simulink model "robot"  (R2024a)
settings: Solver=FixedStepDiscrete  StartTime=0.0  StopTime=inf  FixedStep=0.01  RelTol=1e-3
values from neighbouring files (symbols this model uses):
  markParams = struct()    [markParameters.m]
  mazeForSim = evalin('base',mapVar)    [mySetupRobotSim.m]
  robotParams = struct()    [robotParameters.m]
undefined symbols (not defined in the file or in its folder): D, DiscIntNeverNeededParam, InputPWM, Ts, uDelay, wheelMotorModel, WheelSpeed, xinit, yDelay
libraries: simulink x20, cstblocks x2, simulink_extras x1, mobileRoboticsTrainingLib x1
settings Model: Creator=ngcoya  LastModifiedBy=ngcoya
settings DataIOCC: ExternalInput=maze

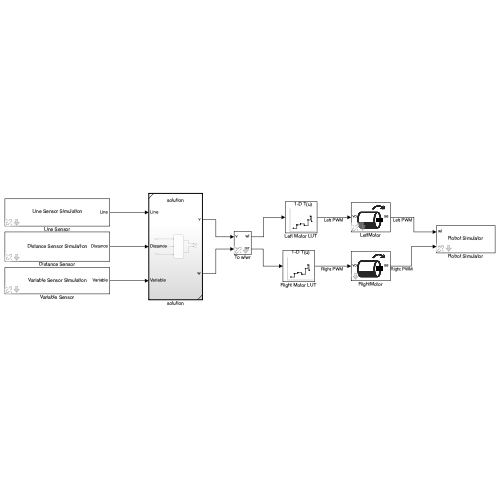
[thumbnail: Simulink's stored preview of the top-level diagram]
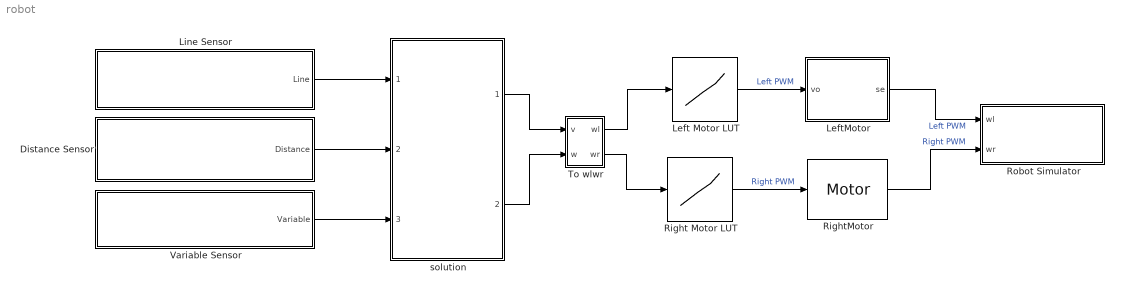
== system robot ==
  Distance Sensor : Subsystem  AncestorBlock=mobileRoboticsTrainingLib/Line Sensor  mask(Line Sensor Simulation){mapVariable=mazeForSim}
      mask prompts: mapVariable "Map Variable"
      mask help: Use a simulation map to compute line sensor values based on robot position and sensor offsets.
      mask Help: web('Line Sensor Simulation.htm')
      mask DialogControl DescTextVar Prompt: Use a simulation map to compute distance sensor values based on robot position and sensor parameters.
      mask DialogControl mapCont Prompt: Map Setup
      mask Display: disp('Distance Sensor Simulation')
  Left Motor LUT : Lookup_n-D  NumberOfTableDimensions=1  BreakpointsForDimension1=WheelSpeed  Table=InputPWM  InterpMethod=Nearest  ExtrapMethod=Clip  InternalRulePriority=Speed  RndMeth=Simplest
  LeftMotor : Subsystem  AncestorBlock=mobileRoboticsTrainingLib/Motor  mask(Motor Model){motorPlant=wheelMotorModel, sensorType=Speed}
      mask prompts: motorPlant "Motor Model"; sensorType "Sensor Type"
      mask help: Use LTI systems to model motors obtained through workflows such as the System Identification App.
      mask Help: web('Motor.htm')
      mask TypeOptions sensorType: Speed | Position
      mask Display:
      | img = imread('motorMask.png');
      | image(img)
  Line Sensor : Subsystem  AncestorBlock=mobileRoboticsTrainingLib/Line Sensor  mask(Line Sensor Simulation){mapVariable=mazeForSim}
      mask prompts: mapVariable "Map Variable"
      mask help: Use a simulation map to compute line sensor values based on robot position and sensor offsets.
      mask Help: web('Line Sensor Simulation.htm')
      mask DialogControl DescTextVar Prompt: Use a simulation map to compute line sensor values based on robot position and sensor parameters.
      mask DialogControl mapCont Prompt: Map Setup
      mask Display: disp('Line Sensor Simulation')
  Right Motor LUT : Lookup_n-D  NumberOfTableDimensions=1  BreakpointsForDimension1=WheelSpeed  Table=InputPWM  InterpMethod=Nearest  ExtrapMethod=Clip  InternalRulePriority=Speed  RndMeth=Simplest
  RightMotor : mobileRoboticsTrainingLib/Motor  motorPlant=wheelMotorModel  sensorType=Speed
      settings: SourceProductName=Mobile Robotics Training Library
  Robot Simulator : Subsystem  Priority=99  AncestorBlock=mobileRoboticsTrainingLib/Robot Simulator  mask(Robot Simulator){mapVar=mazeForSim, startX=100, startY=100, startTheta=0, axleLength=robotParams.axleLength, wheelR=robotParams.wheelR, robustness=False}
      mask prompts: mapVar "Map Variable"; startX "Start X (mm)"; startY "Start Y (mm)"; startTheta "Theta (deg)"; axleLength "Axle Length (mm)"; wheelR "Wheel Radius (mm)"; robustness "Test robustness"
      mask help: Configure robot simulator to use custom simulation maps and simulate closed-loop mobile robotics systems along with appropriate sensor simulation blocks.
      mask init:
      | set_param(bdroot,'SolverType','Fixed-Step');
      | set_param(bdroot,'Solver','FixedStepDiscrete');
      | 
      | if (exist('Ts'))
      |     set_param(bdroot,'FixedStep','Ts');
      | else
      |     set_param(bdroot,'FixedStep','0.01');
      | end
      | 
      | h = findobj('Name','Robot Simulator');
      | if ~isempty(h)
      |     close (h);
      | end
      | mySetupRobotSim();
      mask Help: web('Robot Simulator.htm')
      mask DialogControl mapCont Prompt: Map Setup
      mask DialogControl initPosCont Prompt: Initial Position
      mask DialogControl setPos Prompt: Set position interactively
      mask DialogControl setPos Callback:
      | %% Set starting point
      | setStartingPoint();
      mask DialogControl initOrientation Prompt: Initial Orientation
      mask DialogControl robotCharCont Prompt: Robot Characteristics
      mask DialogControl Robustness Prompt: Code Robustness
      mask Display: disp('Robot Simulator')
  To wlwr : Subsystem  AncestorBlock=mobileRoboticsTrainingLib/To wlwr  mask(To wlwr){axleLength=robotParams.axleLength, wheelR=robotParams.wheelR}
      mask prompts: axleLength "Axle Length (m)"; wheelR "Wheel Radius (m)"
      mask help: Converts robot linear (v) and angular (w) velocities into left (wl) and right (wr) wheel angular velocities using robot parameters.
      mask Help: web('To wlwr.htm')
  Variable Sensor : Subsystem  AncestorBlock=mobileRoboticsTrainingLib/Line Sensor  mask(Line Sensor Simulation){mapVariable=mazeForSim, senType=Line Follow}
      mask prompts: mapVariable "Map Variable"
      mask help: Use a simulation map to compute line sensor values based on robot position and sensor offsets.
      mask Help: web('Line Sensor Simulation.htm')
      mask DialogControl DescTextVar Prompt: Use a simulation map to compute sensor values based on robot position and sensor parameters. Please indacte the operation of the sensor based on the operation of use.
      mask DialogControl mapCont Prompt: Map Setup
      mask DialogControl senCont Prompt: Sensor Characteristics
      mask Display: disp('Variable Sensor Simulation')
  solution : Subsystem  TreatAsAtomicUnit=on  ReferencedSubsystem=solution
  wires:
  Right Motor LUT/1 -> RightMotor/1  "Right PWM"
  Left Motor LUT/1 -> LeftMotor/1(vo)  "Left PWM"
  Line Sensor/1(Line) -> solution/1
  Distance Sensor/1(Distance) -> solution/2
  Variable Sensor/1(Variable) -> solution/3
  To wlwr/1(wl) -> Left Motor LUT/1
  To wlwr/2(wr) -> Right Motor LUT/1
  solution/1 -> To wlwr/1(v)
  solution/2 -> To wlwr/2(w)
  RightMotor/1 -> Robot Simulator/2(wr)  "Right PWM"
  LeftMotor/1(se) -> Robot Simulator/1(wl)  "Left PWM"

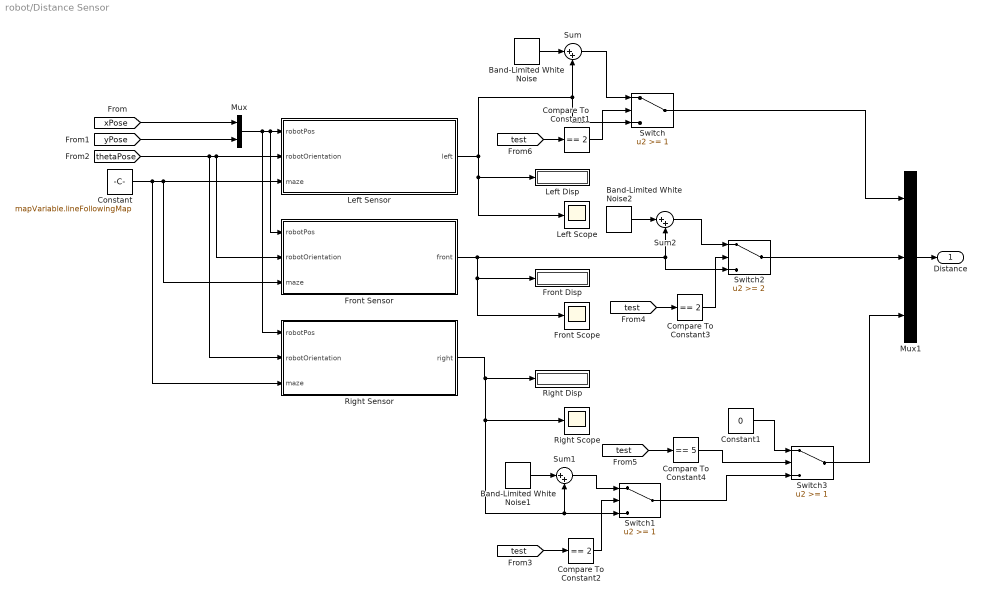
== system robot/Distance Sensor ==
  Band-Limited White Noise : simulink/Sources/Band-Limited White Noise  Cov=[0.1]  Ts=0.1  seed=[23341]
  Band-Limited White Noise1 : simulink/Sources/Band-Limited White Noise  Cov=[0.1]  Ts=0.1  seed=[23341]
  Band-Limited White Noise2 : simulink/Sources/Band-Limited White Noise  Cov=[0.1]  Ts=0.1  seed=[23341]
  Compare To Constant1 : simulink/Logic and Bit Operations/Compare To Constant  relop===  const=2  OutDataTypeStr=boolean
  Compare To Constant2 : simulink/Logic and Bit Operations/Compare To Constant  relop===  const=2  OutDataTypeStr=boolean
  Compare To Constant3 : simulink/Logic and Bit Operations/Compare To Constant  relop===  const=2  OutDataTypeStr=boolean
  Compare To Constant4 : simulink/Logic and Bit Operations/Compare To Constant  relop===  const=5  OutDataTypeStr=boolean
  Constant : Constant  Value=mapVariable.lineFollowingMap
  Constant1 : Constant  Value=0
  Front Disp : Display
  Front Scope : Scope
  Front Sensor : MATLAB Function  TreatAsAtomicUnit=on
  Left Disp : Display
  Left Scope : Scope
  Left Sensor : MATLAB Function  TreatAsAtomicUnit=on
  Mux : Mux  Inputs=2
  Mux1 : Mux  Inputs=3
  Right Disp : Display
  Right Scope : Scope
  Right Sensor : MATLAB Function  TreatAsAtomicUnit=on
  Sum : Sum  Inputs=|++
  Sum1 : Sum  Inputs=|++
  Sum2 : Sum  Inputs=|++
  Switch : Switch  Threshold=1  SaturateOnIntegerOverflow=off  InputSameDT=off
  Switch1 : Switch  Threshold=1  SaturateOnIntegerOverflow=off  InputSameDT=off
  Switch2 : Switch  Threshold=2  SaturateOnIntegerOverflow=off  InputSameDT=off
  Switch3 : Switch  Threshold=1  SaturateOnIntegerOverflow=off  InputSameDT=off
  Distance : Outport
  wires:
  [xPose] -> Mux/1
  [yPose] -> Mux/2
  Left Sensor/1(left) -> Switch/3, Sum/2, Left Scope/1, Left Disp/1
  Front Sensor/1(front) -> Switch2/3, Sum2/2, Front Scope/1, Front Disp/1
  [thetaPose] -> Left Sensor/2(robotOrientation), Front Sensor/2(robotOrientation), Right Sensor/2(robotOrientation)
  Constant/1 -> Right Sensor/3(maze), Front Sensor/3(maze), Left Sensor/3(maze)
  Mux/1 -> Right Sensor/1(robotPos), Front Sensor/1(robotPos), Left Sensor/1(robotPos)
  Right Sensor/1(right) -> Switch1/3, Sum1/2, Right Scope/1, Right Disp/1
  Mux1/1 -> Distance/1
  [test] -> Compare To Constant1/1
  Sum/1 -> Switch/1
  Band-Limited White Noise/1 -> Sum/1
  Sum1/1 -> Switch1/1
  Band-Limited White Noise1/1 -> Sum1/1
  [test] -> Compare To Constant2/1
  Switch1/1 -> Switch3/3
  Switch/1 -> Mux1/1
  [test] -> Compare To Constant3/1
  Sum2/1 -> Switch2/1
  Band-Limited White Noise2/1 -> Sum2/1
  Switch2/1 -> Mux1/2
  Compare To Constant1/1 -> Switch/2
  Compare To Constant2/1 -> Switch1/2
  Compare To Constant3/1 -> Switch2/2
  [test] -> Compare To Constant4/1
  Compare To Constant4/1 -> Switch3/2
  Constant1/1 -> Switch3/1
  Switch3/1 -> Mux1/3

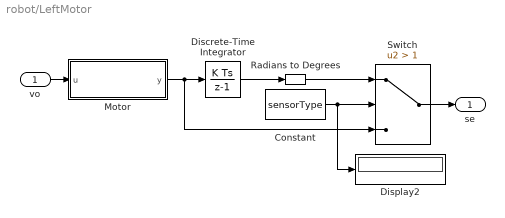
== system robot/LeftMotor ==
  vo : Inport
  Constant : Constant  Value=sensorType
  Discrete-Time Integrator : DiscreteIntegrator  SampleTime=-1  ICPrevOutput=DiscIntNeverNeededParam  ICPrevScaledInput=DiscIntNeverNeededParam
  Display2 : Display
  Motor : Subsystem  AncestorBlock=cstblocks/LTI System  BlockChoice=CSS  mask(LTI Block){sys=motorPlant, IC=[], PadeOrder=0}
      mask prompts: sys "Control:simulink:LTIMaskLabel1"; IC "Control:simulink:LTIMaskLabel2"; PadeOrder "Pade Order (for linearization)"
      mask help: Control:simulink:LTIMaskDescription
      mask init:
      | model = bdroot;
      | df = get_param(model,'dirty');
      | try
      |     [D,uDelay,yDelay,xinit,Ts,sysname] = controllib.internal.blocks.lti.ltimaskData(gcb,sys,IC);
      | catch ME
      |     sysname = '???';
      |     throwAsCaller(MSLException(get_param(gcb,'handle'),ME.identifier,ME.message))
      | end
      | controllib.internal.blocks.lti.ltimaskUpdate(gcb,D,xinit,Ts,PadeOrder)
      | try
      |     % Attempt to modify locked library -> error
      |     set_param(model,'dirty',df)
      | end
      mask Help: eval('helpview(''control'',''ltisystemblock'');')
      mask Callback sys: controllib.internal.blocks.lti.ltimaskCallback(gcb,'System')
      mask DialogControl sys Prompt: LTI system variable
      mask DialogControl IC Prompt: Initial states (state-space only)
      mask Display: disp(sysname)
  Radians to Degrees : simulink_extras/Transformations/Radians to Degrees
  Switch : Switch  Criteria=u2 > Threshold  Threshold=1  SaturateOnIntegerOverflow=off  InputSameDT=off
  se : Outport
  wires:
  Motor/1(y) -> Switch/3, Discrete-Time Integrator/1
  Switch/1 -> se/1
  vo/1 -> Motor/1(u)
  Constant/1 -> Display2/1, Switch/2
  Discrete-Time Integrator/1 -> Radians to Degrees/1
  Radians to Degrees/1 -> Switch/1

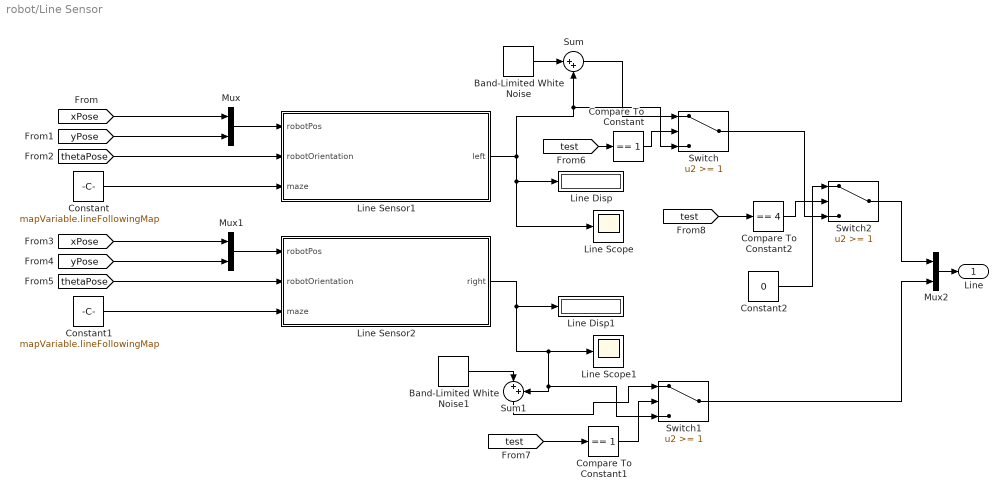
== system robot/Line Sensor ==
  Band-Limited White Noise : simulink/Sources/Band-Limited White Noise  Cov=[0.1]  Ts=0.1  seed=[23341]
  Band-Limited White Noise1 : simulink/Sources/Band-Limited White Noise  Cov=[0.1]  Ts=0.1  seed=[23341]
  Compare To Constant : simulink/Logic and Bit Operations/Compare To Constant  relop===  const=1  OutDataTypeStr=boolean
  Compare To Constant1 : simulink/Logic and Bit Operations/Compare To Constant  relop===  const=1  OutDataTypeStr=boolean
  Compare To Constant2 : simulink/Logic and Bit Operations/Compare To Constant  relop===  const=4  OutDataTypeStr=boolean
  Constant : Constant  Value=mapVariable.lineFollowingMap
  Constant1 : Constant  Value=mapVariable.lineFollowingMap
  Constant2 : Constant  Value=0
  Line Disp : Display
  Line Disp1 : Display
  Line Scope : Scope
  Line Scope1 : Scope
  Line Sensor1 : MATLAB Function  TreatAsAtomicUnit=on
  Line Sensor2 : MATLAB Function  TreatAsAtomicUnit=on
  Mux : Mux  Inputs=2
  Mux1 : Mux  Inputs=2
  Mux2 : Mux  Inputs=2
  Sum : Sum  Inputs=|++
  Sum1 : Sum  Inputs=|++
  Switch : Switch  Threshold=1  SaturateOnIntegerOverflow=off  InputSameDT=off
  Switch1 : Switch  Threshold=1  SaturateOnIntegerOverflow=off  InputSameDT=off
  Switch2 : Switch  Threshold=1  SaturateOnIntegerOverflow=off  InputSameDT=off
  Line : Outport
  wires:
  [yPose] -> Mux/2
  [xPose] -> Mux/1
  Line Sensor1/1(left) -> Switch/3, Sum/2, Line Scope/1, Line Disp/1
  [thetaPose] -> Line Sensor1/2(robotOrientation)
  Mux/1 -> Line Sensor1/1(robotPos)
  Constant/1 -> Line Sensor1/3(maze)
  Constant1/1 -> Line Sensor2/3(maze)
  [yPose] -> Mux1/2
  [thetaPose] -> Line Sensor2/2(robotOrientation)
  [xPose] -> Mux1/1
  Line Sensor2/1(right) -> Line Scope1/1, Switch1/3, Sum1/2, Line Disp1/1
  Mux1/1 -> Line Sensor2/1(robotPos)
  Mux2/1 -> Line/1
  [test] -> Compare To Constant/1
  Band-Limited White Noise/1 -> Sum/1
  Sum/1 -> Switch/1
  [test] -> Compare To Constant1/1
  Sum1/1 -> Switch1/1
  Band-Limited White Noise1/1 -> Sum1/1
  Switch1/1 -> Mux2/2
  Compare To Constant/1 -> Switch/2
  Compare To Constant1/1 -> Switch1/2
  [test] -> Compare To Constant2/1
  Compare To Constant2/1 -> Switch2/2
  Switch/1 -> Switch2/3
  Switch2/1 -> Mux2/1
  Constant2/1 -> Switch2/1

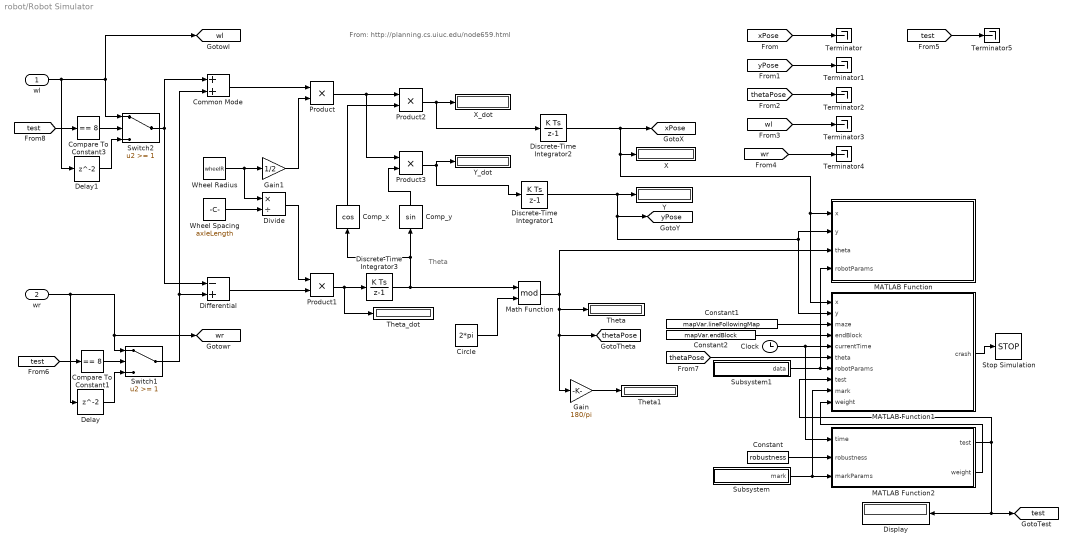
== system robot/Robot Simulator ==
  note: Theta
  note: From: http://planning.cs.uiuc.edu/node659.html
  wl : Inport
  wr : Inport  Port=2
  Circle : Constant  Value=2*pi
  Clock : Clock
  Common Mode : Sum
  Comp_x : Trigonometry  Operator=cos
  Comp_y : Trigonometry
  Compare To Constant1 : simulink/Logic and Bit Operations/Compare To Constant  relop===  const=8  OutDataTypeStr=boolean
  Compare To Constant3 : simulink/Logic and Bit Operations/Compare To Constant  relop===  const=8  OutDataTypeStr=boolean
  Constant : Constant  Value=robustness
  Constant1 : Constant  Value=mapVar.lineFollowingMap
  Constant2 : Constant  Value=mapVar.endBlock
  Delay : Delay
  Delay1 : Delay
  Differential : Sum  Inputs=-+
  Discrete-Time Integrator1 : DiscreteIntegrator  InitialCondition=startY  SampleTime=-1  ICPrevOutput=DiscIntNeverNeededParam  ICPrevScaledInput=DiscIntNeverNeededParam
  Discrete-Time Integrator2 : DiscreteIntegrator  InitialCondition=startX  SampleTime=-1  ICPrevOutput=DiscIntNeverNeededParam  ICPrevScaledInput=DiscIntNeverNeededParam
  Discrete-Time Integrator3 : DiscreteIntegrator  InitialCondition=startTheta  SampleTime=-1  ICPrevOutput=DiscIntNeverNeededParam  ICPrevScaledInput=DiscIntNeverNeededParam
  Display : Display
  Divide : Product  Inputs=*/
  Gain : Gain  Gain=180/pi
  Gain1 : Gain  Gain=1/2
  MATLAB Function : MATLAB Function  TreatAsAtomicUnit=on
  MATLAB Function1 : MATLAB Function  TreatAsAtomicUnit=on
  MATLAB Function2 : MATLAB Function  TreatAsAtomicUnit=on
  Math Function : Math  Operator=mod  SignedPower=on
  Product{,1..3} (4 alike) : Product  RndMeth=Zero
  Stop Simulation : Stop
  Subsystem : Subsystem
  Subsystem1 : Subsystem
  Switch1 : Switch  Threshold=1  SaturateOnIntegerOverflow=off  InputSameDT=off
  Switch2 : Switch  Threshold=1  SaturateOnIntegerOverflow=off  InputSameDT=off
  Terminator{,1..5} (6 alike) : Terminator
  Theta : Display
  Theta1 : Display
  Theta_dot : Display
  Wheel Radius : Constant  Value=wheelR
  Wheel Spacing : Constant  Value=axleLength
  X : Display
  X_dot : Display
  Y : Display
  Y_dot : Display
  tag scope: test=global, thetaPose=global, wl=global, wr=global, xPose=global, yPose=global
  wires:
  [wr] -> Terminator4/1
  [wl] -> Terminator3/1
  Math Function/1 -> MATLAB Function/3(theta), Gain/1, [thetaPose], Theta/1
  Differential/1 -> Product1/2
  Comp_y/1 -> Product3/2
  Discrete-Time Integrator2/1 -> MATLAB Function1/1(x), MATLAB Function/1(x), X/1, [xPose]
  Product3/1 -> Discrete-Time Integrator1/1, Y_dot/1
  Discrete-Time Integrator1/1 -> MATLAB Function1/2(y), MATLAB Function/2(y), [yPose], Y/1
  Divide/1 -> Product1/1
  Discrete-Time Integrator3/1 -> Math Function/1, Comp_x/1, Comp_y/1
  Comp_x/1 -> Product2/2
  Product1/1 -> Discrete-Time Integrator3/1, Theta_dot/1
  Wheel Radius/1 -> Divide/1, Gain1/1
  Wheel Spacing/1 -> Divide/2
  Product2/1 -> Discrete-Time Integrator2/1, X_dot/1
  Gain1/1 -> Product/2
  Common Mode/1 -> Product/1
  Product/1 -> Product3/1, Product2/1
  Circle/1 -> Math Function/2
  [xPose] -> Terminator/1
  [yPose] -> Terminator1/1
  [thetaPose] -> Terminator2/1
  Constant1/1 -> MATLAB Function1/3(maze)
  Constant2/1 -> MATLAB Function1/4(endBlock)
  MATLAB Function1/1(crash) -> Stop Simulation/1
  wl/1 -> Delay1/1, Switch2/1, [wl]
  wr/1 -> Delay/1, [wr], Switch1/1
  Clock/1 -> MATLAB Function2/1(time), MATLAB Function1/5(currentTime)
  Constant/1 -> MATLAB Function2/2(robustness)
  MATLAB Function2/1(test) -> Display/1, [test], MATLAB Function1/8(test)
  Subsystem/1(mark) -> MATLAB Function1/9(mark), MATLAB Function2/3(markParams)
  [test] -> Terminator5/1
  Delay1/1 -> Switch2/3
  Compare To Constant3/1 -> Switch2/2
  [test] -> Compare To Constant3/1
  [test] -> Compare To Constant1/1
  Delay/1 -> Switch1/3
  Compare To Constant1/1 -> Switch1/2
  Switch2/1 -> Common Mode/1, Differential/1
  Switch1/1 -> Common Mode/2, Differential/2
  Subsystem1/1(data) -> MATLAB Function/4(robotParams), MATLAB Function1/7(robotParams)
  [thetaPose] -> MATLAB Function1/6(theta)
  MATLAB Function2/2(weight) -> MATLAB Function1/10(weight)
  Gain/1 -> Theta1/1

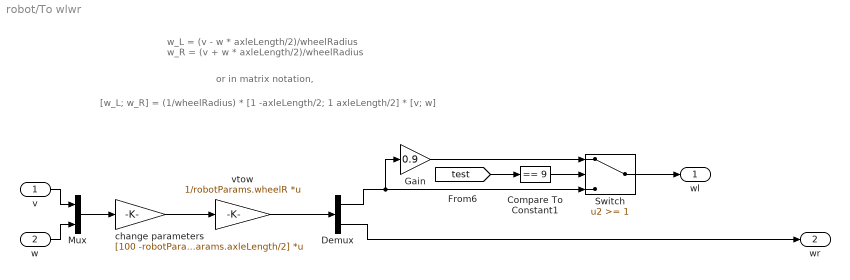
== system robot/To wlwr ==
  note: or in matrix notation,
  note: w_L  = (v - w * axleLength/2)/wheelRadius
      | w_R = (v + w * axleLength/2)/wheelRadius
  note: [w_L; w_R] = (1/wheelRadius) * [1 -axleLength/2; 1 axleLength/2] * [v; w]
  v : Inport
  w : Inport  Port=2
  Compare To Constant1 : simulink/Logic and Bit Operations/Compare To Constant  relop===  const=9  OutDataTypeStr=boolean
  Demux : Demux  Outputs=2
  Gain : Gain  Gain=0.9
  Mux : Mux  Inputs=2
  Switch : Switch  Threshold=1  SaturateOnIntegerOverflow=off  InputSameDT=off
  change parameters : Gain  Gain=[100 -robotParams.axleLength/2;100 robotParams.axleLength/2]  Multiplication=Matrix(K*u)
  vtow : Gain  Gain=1/robotParams.wheelR  Multiplication=Matrix(K*u)
  wl : Outport
  wr : Outport  Port=2
  wires:
  vtow/1 -> Demux/1
  change parameters/1 -> vtow/1
  Demux/2 -> wr/1
  v/1 -> Mux/1
  w/1 -> Mux/2
  Mux/1 -> change parameters/1
  [test] -> Compare To Constant1/1
  Compare To Constant1/1 -> Switch/2
  Demux/1 -> Switch/3, Gain/1
  Switch/1 -> wl/1
  Gain/1 -> Switch/1

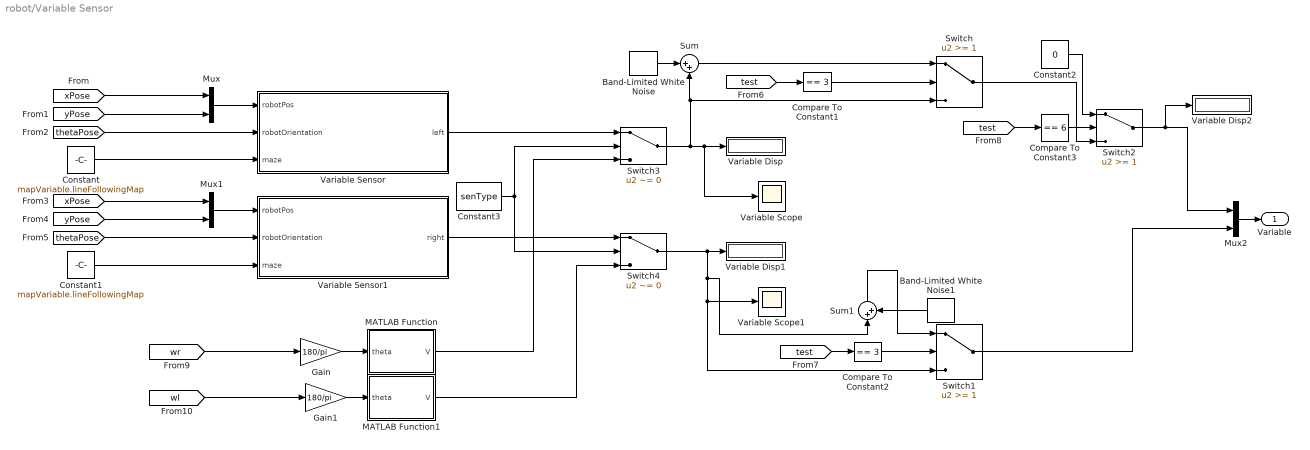
== system robot/Variable Sensor ==
  Band-Limited White Noise : simulink/Sources/Band-Limited White Noise  Cov=[0.1]  Ts=0.1  seed=[23341]
  Band-Limited White Noise1 : simulink/Sources/Band-Limited White Noise  Cov=[0.1]  Ts=0.1  seed=[23341]
  Compare To Constant1 : simulink/Logic and Bit Operations/Compare To Constant  relop===  const=3  OutDataTypeStr=boolean
  Compare To Constant2 : simulink/Logic and Bit Operations/Compare To Constant  relop===  const=3  OutDataTypeStr=boolean
  Compare To Constant3 : simulink/Logic and Bit Operations/Compare To Constant  relop===  const=6  OutDataTypeStr=boolean
  Constant : Constant  Value=mapVariable.lineFollowingMap
  Constant1 : Constant  Value=mapVariable.lineFollowingMap
  Constant2 : Constant  Value=0
  Constant3 : Constant  Value=senType
  Gain : Gain  Gain=180/pi
  Gain1 : Gain  Gain=180/pi
  MATLAB Function : MATLAB Function  TreatAsAtomicUnit=on
  MATLAB Function1 : MATLAB Function  TreatAsAtomicUnit=on
  Mux : Mux  Inputs=2
  Mux1 : Mux  Inputs=2
  Mux2 : Mux  Inputs=2
  Sum : Sum  Inputs=|++
  Sum1 : Sum  Inputs=|++
  Switch : Switch  Threshold=1  SaturateOnIntegerOverflow=off  InputSameDT=off
  Switch1 : Switch  Threshold=1  SaturateOnIntegerOverflow=off  InputSameDT=off
  Switch2 : Switch  Threshold=1  SaturateOnIntegerOverflow=off  InputSameDT=off
  Switch3 : Switch  Criteria=u2 ~= 0  SaturateOnIntegerOverflow=off  InputSameDT=off
  Switch4 : Switch  Criteria=u2 ~= 0  SaturateOnIntegerOverflow=off  InputSameDT=off
  Variable Disp : Display
  Variable Disp1 : Display
  Variable Disp2 : Display
  Variable Scope : Scope
  Variable Scope1 : Scope
  Variable Sensor : MATLAB Function  TreatAsAtomicUnit=on
  Variable Sensor1 : MATLAB Function  TreatAsAtomicUnit=on
  Variable : Outport
  wires:
  Constant/1 -> Variable Sensor/3(maze)
  [yPose] -> Mux/2
  [thetaPose] -> Variable Sensor/2(robotOrientation)
  Mux/1 -> Variable Sensor/1(robotPos)
  [xPose] -> Mux/1
  Mux1/1 -> Variable Sensor1/1(robotPos)
  [yPose] -> Mux1/2
  [xPose] -> Mux1/1
  [thetaPose] -> Variable Sensor1/2(robotOrientation)
  Constant1/1 -> Variable Sensor1/3(maze)
  Mux2/1 -> Variable/1
  [test] -> Compare To Constant1/1
  Sum/1 -> Switch/1
  Band-Limited White Noise/1 -> Sum/1
  Switch/1 -> Switch2/3
  Sum1/1 -> Switch1/1
  [test] -> Compare To Constant2/1
  Switch1/1 -> Mux2/2
  Compare To Constant1/1 -> Switch/2
  Compare To Constant2/1 -> Switch1/2
  Compare To Constant3/1 -> Switch2/2
  [test] -> Compare To Constant3/1
  Constant2/1 -> Switch2/1
  Variable Sensor/1(left) -> Switch3/1
  Switch3/1 -> Variable Disp/1, Variable Scope/1, Switch/3, Sum/2
  Constant3/1 -> Switch3/2, Switch4/2
  Switch4/1 -> Variable Disp1/1, Switch1/3, Variable Scope1/1, Sum1/1
  Band-Limited White Noise1/1 -> Sum1/2
  [wr] -> Gain/1
  Gain/1 -> MATLAB Function/1(theta)
  Gain1/1 -> MATLAB Function1/1(theta)
  [wl] -> Gain1/1
  MATLAB Function1/1(V) -> Switch4/3
  MATLAB Function/1(V) -> Switch3/3
  Variable Sensor1/1(right) -> Switch4/1
  Switch2/1 -> Variable Disp2/1, Mux2/1

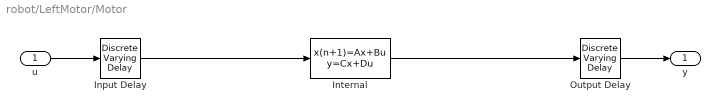
== system robot/LeftMotor/Motor ==
  u : Inport  PortDimensions=1  SampleTime=Ts
  Input Delay : cstblocks/Linear Parameter Varying/Discrete Varying Delay  Td=uDelay  TdMax=max(uDelay)  TdFixed=1  u0=0  Ts=Ts  PreventDirectFeedthrough=off
  Internal : DiscreteStateSpace  A=D.a  B=D.b  C=D.c  D=D.d  InitialCondition=xinit  SampleTime=Ts
  Output Delay : cstblocks/Linear Parameter Varying/Discrete Varying Delay  Td=yDelay  TdMax=max(yDelay)  TdFixed=1  u0=0  Ts=-1  PreventDirectFeedthrough=off
  y : Outport  InitialOutput=0  VectorParamsAs1DForOutWhenUnconnected=off
  wires:
  u/1 -> Input Delay/1
  Output Delay/1 -> y/1
  Input Delay/1 -> Internal/1
  Internal/1 -> Output Delay/1

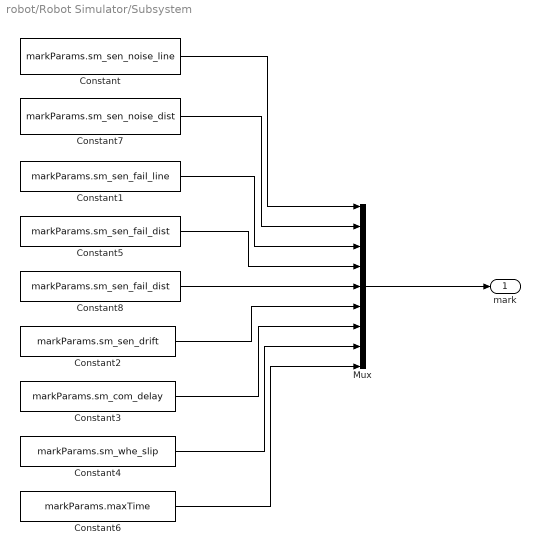
== system robot/Robot Simulator/Subsystem ==
  Constant : Constant  Value=markParams.sm_sen_noise_line
  Constant1 : Constant  Value=markParams.sm_sen_fail_line
  Constant2 : Constant  Value=markParams.sm_sen_drift
  Constant3 : Constant  Value=markParams.sm_com_delay
  Constant4 : Constant  Value=markParams.sm_whe_slip
  Constant5 : Constant  Value=markParams.sm_sen_fail_dist
  Constant6 : Constant  Value=markParams.maxTime
  Constant7 : Constant  Value=markParams.sm_sen_noise_dist
  Constant8 : Constant  Value=markParams.sm_sen_fail_dist
  Mux : Mux  Inputs=9
  mark : Outport
  wires:
  Constant/1 -> Mux/1
  Constant1/1 -> Mux/3
  Constant2/1 -> Mux/6
  Constant3/1 -> Mux/7
  Constant4/1 -> Mux/8
  Mux/1 -> mark/1
  Constant6/1 -> Mux/9
  Constant7/1 -> Mux/2
  Constant5/1 -> Mux/4
  Constant8/1 -> Mux/5

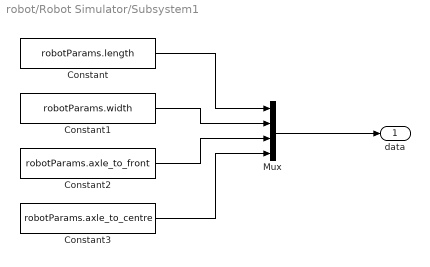
== system robot/Robot Simulator/Subsystem1 ==
  Constant : Constant  Value=robotParams.length
  Constant1 : Constant  Value=robotParams.width
  Constant2 : Constant  Value=robotParams.axle_to_front
  Constant3 : Constant  Value=robotParams.axle_to_centre
  Mux : Mux
  data : Outport
  wires:
  Constant/1 -> Mux/1
  Constant1/1 -> Mux/2
  Mux/1 -> data/1
  Constant2/1 -> Mux/3
  Constant3/1 -> Mux/4

== matlab function robot/Robot Simulator/MATLAB Function2 ==
  data: time input; robustness input; test output; markParams input; weight output
function [test, weight] = setTest(time, robustness, markParams)
    test = 0;
    weight = zeros(1, 8);
    persistent markArray total maxTime;

    if isempty(markArray) && robustness                                     % Get struct from base workspace
        rawArray = [ ...
            markParams(1), ...
            markParams(2), ...
            markParams(3), ...
            markParams(4), ...
            markParams(5), ...
            markParams(6), ...
            markParams(7), ...
            markParams(8) ...
        ];
        maxTime = markParams(9);
        total = sum(rawArray);
        markArray = zeros(1, length(rawArray));
        cumulative = 0;
        for n = 1:length(rawArray)
            cumulative = cumulative + rawArray(n);
            markArray(n) = (cumulative / total) * 100;
        end
    end
    if robustness && ~isempty(maxTime)
        currentPercent = (time / maxTime) * 100;
        if currentPercent < markArray(1)
            test = 1;
            weight(1) = round(currentPercent * 100/markArray(1));
        elseif currentPercent < markArray(2)
            test = 2;
            weight(2) = round(currentPercent * 100/markArray(2));
        elseif currentPercent < markArray(3)
            test = 3;
            weight(3) = round(currentPercent * 100/markArray(3));
        elseif currentPercent < markArray(4)
            test = 4;
            weight(4) = round(currentPercent * 100/markArray(4));
        elseif currentPercent < markArray(5)
            test = 5;
            weight(5) = round(currentPercent * 100/markArray(5));
        elseif currentPercent < markArray(6)
            test = 6;
            weight(6) = round(currentPercent * 100/markArray(6));
        elseif currentPercent < markArray(7)
            test = 7;
            weight(7) = round(currentPercent * 100/markArray(7));
        elseif currentPercent < markArray(8)
            test = 8;
            weight(8) = round(currentPercent * 100/markArray(8));
        end
    end

== matlab function robot/Variable Sensor/MATLAB Function ==
  data: theta input; V output
function V = voltage(theta)

theta_mod = mod(theta, 360);

angles = mod(theta_mod - 1 : 1 : theta_mod + 1, 360);                           % Field of view: ±1 degrees

segment_indices = floor(angles / (360/20));                                     % Determine segment index

is_white = mod(segment_indices, 2) == 0;                                        % White segments = even indices

white_fraction = sum(is_white) / length(is_white);                              % Fraction of white area

black_fraction = 1 - white_fraction;                                            % Fraction of black area



R = 0.8 * white_fraction + 0.05 * black_fraction;
E_avg = 851.7;
E_eff = R * E_avg;
V_oc = 0.42;
V = V_oc * E_eff;

== matlab function robot/Variable Sensor/MATLAB Function1 ==
  data: theta input; V output
function V = voltage(theta)

theta_mod = mod(theta, 360);

angles = mod(theta_mod - 12 : 1 : theta_mod + 12, 360);                         % Field of view: ±12 degrees

segment_indices = floor(angles / 18);                                           % Determine segment index

is_white = mod(segment_indices, 2) == 0;                                        % White segments = even indices

white_fraction = sum(is_white) / length(is_white);                              % Fraction of white area

black_fraction = sum(is_white) / length(is_white);                              % Fraction of black area



R = 0.8 * white_fraction + 0.05 * black_fraction;
E_avg = 7.98;
E_eff = R * E_avg;
V_oc = 0.42;
V = V_oc * E_eff;

== matlab function robot/Robot Simulator/MATLAB Function ==
  data: x input; y input; theta input; robotParams input
function plotRobot(x, y, theta, robotParams)
    coder.extrinsic('imread', 'image', 'set', 'drawnow', 'evalin');
    persistent plotHandle robotImg alpha;
    degTheta = rad2deg(theta);
    if isempty(robotImg)
        [robotImg, ~, alpha] = imread('mouse_image.png'); % Load a PNG image with transparent background (or JPG)
    end
    
    axleOffset = robotParams(4);
    centreX = x - axleOffset * cos(theta);
    centreY = y - axleOffset * sin(theta);

    rotatedImg = imrotate(robotImg, -degTheta, 'bilinear', 'crop');
    rotatedAlpha = imrotate(alpha, -degTheta, 'bilinear', 'crop');

    halfSize = 147/2;
    bounds = [centreX-halfSize, centreX+halfSize, centreY-halfSize, centreY+halfSize];
    
     if isempty(plotHandle)
        plotHandle = evalin("base", "plotHandle");
    else
        set(plotHandle, 'CData', rotatedImg, ...
                       'XData', bounds(1:2), ...
                       'YData', bounds(3:4), ...
                       'AlphaData', rotatedAlpha);
    end
    
    drawnow('limitrate', 'nocallbacks');
end

== matlab function robot/Distance Sensor/Left Sensor ==
  data: robotPos input; left output; robotOrientation input; maze input
function left = leftSensor(robotPos, robotOrientation, maze)
    x = robotPos(1) + 21 * cos(robotOrientation);
    y = robotPos(2) + 21 * sin(robotOrientation);
    maxRange = 2000;
    
    left = maxRange;
    for t = 1:maxRange
        xNext = round(x + t * sin(robotOrientation));
        yNext = round(y - t * cos(robotOrientation));

        if xNext > 0 && xNext < size(maze,1) && yNext > 0 && yNext < size(maze,2)
            if maze(yNext, xNext) == 1
                left = t;
                break;
            end
        end
    end
end
%{
function left = leftSensor(robotPos, robotOrientation, maze)
    % Precompute trigonometric functions once
    cosTheta = cos(robotOrientation);
    sinTheta = sin(robotOrientation);
    
    % Initial sensor position
    x = robotPos(1) + 21 * cosTheta;
    y = robotPos(2) + 21 * sinTheta;
    
    % Direction vector components
    dx = sinTheta;
    dy = -cosTheta;
    
    % Maze boundaries
    [rows, cols] = size(maze);
    maxRange = min(2000, max(rows, cols));  % Don't exceed maze dimensions
    
    % Vectorized approach
    t_values = 1:maxRange;
    x_coords = round(x + t_values * dx);
    y_coords = round(y + t_values * dy);
    
    % Find valid indices within maze boundaries
    valid_idx = (x_coords >= 1 & x_coords <= cols & ...
                y_coords >= 1 & y_coords <= rows);
    
    % Check for obstacles only at valid positions
    obstacle_found = false;
    left = 2000;
    for t = 1:maxRange
        if valid_idx(t)
            if maze(y_coords(t), x_coords(t)) == 1
                left = t;
                obstacle_found = true;
                break;
            end
        else
            % Exit if we're out of bounds
            left = t;
            obstacle_found = true;
            break;
        end
    end
    
    if ~obstacle_found
        left = maxRange;
    end
end
%}

== matlab function robot/Distance Sensor/Front Sensor ==
  data: robotPos input; front output; robotOrientation input; maze input
function front = frontSensor(robotPos, robotOrientation, maze)
    x = robotPos(1);
    y = robotPos(2);
    maxRange = 2000;
    
    front = maxRange;
    for t = 1:maxRange
        xNext = round(x + t * cos(robotOrientation));
        yNext = round(y + t * sin(robotOrientation));


        if xNext > 0 && xNext < size(maze,1) && yNext > 0 && yNext < size(maze,2)
            if maze(yNext, xNext) == 1
                front = round(sqrt((xNext - x)^2 + (y - yNext)^2) - 21);
                break;
            end
        end
    end
end

== matlab function robot/Distance Sensor/Right Sensor ==
  data: robotPos input; right output; robotOrientation input; maze input
function right = rightSensor(robotPos, robotOrientation, maze)
    x = robotPos(1) + 21 * cos(robotOrientation);
    y = robotPos(2) + 21 * sin(robotOrientation);
    maxRange = 2000;

    right = maxRange;
    for t = 1:maxRange
        xNext = round(x - t * sin(robotOrientation));
        yNext = round(y + t * cos(robotOrientation));


        if xNext > 0 && xNext < size(maze,1) && yNext > 0 && yNext < size(maze,2)
            if maze(yNext, xNext) == 1
                right = round(sqrt((xNext - x)^2 + (y - yNext)^2) - 7);
                break;
            end
        end
    end
end

== matlab function robot/Line Sensor/Line Sensor1 ==
  data: robotPos input; left output; robotOrientation input; maze input
function left = lineSensor(robotPos, robotOrientation, maze)
    persistent height width idx r;
    left = 0;

    if isempty(idx)                                 %constant
        [height, width] = size(maze);
        r = 10;
        idx = 1;
    end

    x = robotPos(1) + 11 * cos(robotOrientation);   %Sensor axle pos from x,y
    y = robotPos(2) + 11 * sin(robotOrientation);

    x = x + 5 * sin(robotOrientation);              %Sensor pos from axle
    y = y - 5 * cos(robotOrientation);

    c1x = x - 2 * sin(robotOrientation);            %Centre x and y positions of effective radius
    c1y = y + 2 * sin(robotOrientation);
    c2x = x + 2 * sin(robotOrientation);
    c2y = y - 2 * sin(robotOrientation);

    xMin = max(1, floor(x - 1.5*r));                    %Box space
    xMax = min(width, ceil(x + 1.5*r));
    yMin = max(1, floor(y - 1.5*r));
    yMax = min(height, ceil(y + 1.5*r));
    R = 0;
    count = 0;
    for xi = xMin:xMax
        for yi = yMin:yMax
                value = double(maze(yi, xi));
            if (c1x - xi)^2 + (c1y - yi)^2 <= r^2       %less than circle radius
                count = count + 1;
                if value == 2
                    R = R + 0.05;
                else
                    R = R + 0.3;
                end
            end
            if (c2x - xi)^2 + (c2y - yi)^2 <= r^2       %less than circle radius
                count = count + 1;
                if value == 2
                    R = R + 0.05;
                else
                    R = R + 0.3;
                end
            end
        end
    end
    R = R/count;
    E_avg = 7.98;
    E_eff = R * E_avg;
    V_oc = 0.42;
    left = V_oc * E_eff;
end

== matlab function robot/Variable Sensor/Variable Sensor ==
  data: robotPos input; left output; robotOrientation input; maze input
function left = lineSensor(robotPos, robotOrientation, maze)
    persistent height width idx r;
    left = 0;

    if isempty(idx)                                 %constant
        [height, width] = size(maze);
        r = 10;
        idx = 1;
    end

    x = robotPos(1) + 11 * cos(robotOrientation);   %Sensor axle pos from x,y
    y = robotPos(2) + 11 * sin(robotOrientation);

    x = x + 35 * sin(robotOrientation);             %Sensor pos from axle
    y = y - 35 * cos(robotOrientation);

    c1x = x + 2 * sin(robotOrientation);            %Centre x and y positions of effective radius
    c1y = y - 2 * sin(robotOrientation);
    c2x = x - 2 * sin(robotOrientation);
    c2y = y + 2 * sin(robotOrientation);

    xMin = max(1, floor(x - 1.5*r));                    %Box space
    xMax = min(width, ceil(x + 1.5*r));
    yMin = max(1, floor(y - 1.5*r));
    yMax = min(height, ceil(y + 1.5*r));
    R = 0;
    count = 0;
    for xi = xMin:xMax
        for yi = yMin:yMax
                value = double(maze(yi, xi));
            if (c1x - xi)^2 + (c1y - yi)^2 <= r^2       %less than circle radius
                count = count + 1;
                if value == 2
                    R = R + 0.05;
                else
                    R = R + 0.3;
                end
            end
            if (c2x - xi)^2 + (c2y - yi)^2 <= r^2       %less than circle radius
                count = count + 1;
                if value == 2
                    R = R + 0.05;
                else
                    R = R + 0.3;
                end
            end
        end
    end
    R = R/count;
    E_avg = 7.98;
    E_eff = R * E_avg;
    V_oc = 0.42;
    left = V_oc * E_eff;
end

== matlab function robot/Line Sensor/Line Sensor2 ==
  data: robotPos input; right output; robotOrientation input; maze input
function right = lineSensor(robotPos, robotOrientation, maze)
    persistent height width idx r;
    right = 0;

    if isempty(idx)                                 %constant
        [height, width] = size(maze);
        r = 10;
        idx = 1;
    end

    x = robotPos(1) + 11 * cos(robotOrientation);   %Sensor axle pos from x,y
    y = robotPos(2) + 11 * sin(robotOrientation);

    x = x - 5 * sin(robotOrientation);              %Sensor pos from axle
    y = y + 5 * cos(robotOrientation);

    c1x = x - 2 * sin(robotOrientation);            %Centre x and y positions of effective radius
    c1y = y + 2 * sin(robotOrientation);
    c2x = x + 2 * sin(robotOrientation);
    c2y = y - 2 * sin(robotOrientation);

    xMin = max(1, floor(x - 1.5*r));                    %Box space
    xMax = min(width, ceil(x + 1.5*r));
    yMin = max(1, floor(y - 1.5*r));
    yMax = min(height, ceil(y + 1.5*r));
    R = 0;
    count = 0;
    for xi = xMin:xMax
        for yi = yMin:yMax
                value = double(maze(yi, xi));
            if (c1x - xi)^2 + (c1y - yi)^2 <= r^2       %less than circle radius
                count = count + 1;
                if value == 2
                    R = R + 0.05;
                else
                    R = R + 0.3;
                end
            end
            if (c2x - xi)^2 + (c2y - yi)^2 <= r^2       %less than circle radius
                count = count + 1;
                if value == 2
                    R = R + 0.05;
                else
                    R = R + 0.3;
                end
            end
        end
    end
    R = R/count;
    E_avg = 7.98;
    E_eff = R * E_avg;
    V_oc = 0.42;
    right = V_oc * E_eff;
end

== matlab function robot/Variable Sensor/Variable Sensor1 ==
  data: robotPos input; right output; robotOrientation input; maze input
function right = lineSensor(robotPos, robotOrientation, maze)
    persistent height width idx r;
    right = 0;

    if isempty(idx)                                 %constant
        [height, width] = size(maze);
        r = 10;
        idx = 1;
    end

    x = robotPos(1) + 11 * cos(robotOrientation);   %Sensor axle pos from x,y
    y = robotPos(2) + 11 * sin(robotOrientation);

    x = x - 35 * sin(robotOrientation);         %Sensor pos from axle
    y = y + 35 * cos(robotOrientation);

    c1x = x - 2 * sin(robotOrientation);            %Centre x and y positions of effective radius
    c1y = y + 2 * sin(robotOrientation);
    c2x = x + 2 * sin(robotOrientation);
    c2y = y - 2 * sin(robotOrientation);

    xMin = max(1, floor(x - 1.5*r));                    %Box space
    xMax = min(width, ceil(x + 1.5*r));
    yMin = max(1, floor(y - 1.5*r));
    yMax = min(height, ceil(y + 1.5*r));
    R = 0;
    count = 0;
    for xi = xMin:xMax
        for yi = yMin:yMax
                value = double(maze(yi, xi));
            if (c1x - xi)^2 + (c1y - yi)^2 <= r^2       %less than circle radius
                count = count + 1;
                if value == 2
                    R = R + 0.05;
                else
                    R = R + 0.3;
                end
            end
            if (c2x - xi)^2 + (c2y - yi)^2 <= r^2       %less than circle radius
                count = count + 1;
                if value == 2
                    R = R + 0.05;
                else
                    R = R + 0.3;
                end
            end
        end
    end
    R = R/count;
    E_avg = 7.98;
    E_eff = R * E_avg;
    V_oc = 0.42;
    right = V_oc * E_eff;
end

== matlab function robot/Robot Simulator/MATLAB Function1 ==
  data: x input; y input; maze input; endBlock input; crash output; currentTime input; theta input; robotParams input; test input; mark input; weight input
function crash = runFunction(x, y, maze, endBlock, currentTime, theta, robotParams, test, mark, weight)
    persistent startTime endTime exploration idx simulationParams;
    crash = false;
    degTheta = rad2deg(theta);
    if isempty(startTime)
        startTime = 0;
        endTime = 0;
    end
    if isempty(idx)
        idx = 1;
        exploration = repmat(' ', 250, 5);
        exploration(1,:) = char('00x00');
        simulationParams = struct();
        simulationParams.finishTime = 0;
        simulationParams.explorationArray = exploration;
        simulationParams.sen_noise_line = 0;
        simulationParams.sen_noise_dist = 0;
        simulationParams.sen_drift = 0;
        simulationParams.sen_fail_line = 0;
        simulationParams.sen_fail_dist = 0;
        simulationParams.sen_fail_var = 0;
        simulationParams.com_delay = 0;
        simulationParams.whe_slip = 0;
    end
    
    if currentTime >= 3
        crash = true;
    end

    x = round(x);
    y = round(y);

    block = sprintf('%02dX%02d', int16(floor(x/200)), int16(floor(y/200)));
    lastBlock = exploration(idx,:);
    if ~isequal(lastBlock, block)
        idx = idx + 1;
        exploration(idx,:) = block;
        simulationParams.explorationArray = exploration;
    end
    
    if x > 0 && y > 0 && x < size(maze, 2) && y < size(maze,1)
        centreX = x - robotParams(4) * cos(theta);
        centreY = y - robotParams(4) * sin(theta);
        halfL = robotParams(1) / 2;
        halfW = robotParams(2) / 2;

        cornersLocal = [...
        -halfL, -halfW;
        -halfL,  halfW;
         halfL,  halfW;
         halfL, -halfW];

        R = [cos(theta), -sin(theta); sin(theta), cos(theta)];

        cornersGlobal = (R * cornersLocal')';
        cornersGlobal(:,1) = cornersGlobal(:,1) + centreX;
        cornersGlobal(:,2) = cornersGlobal(:,2) + centreY;

        minX = floor(min(cornersGlobal(:,1)));
        maxX = ceil(max(cornersGlobal(:,1)));
        minY = floor(min(cornersGlobal(:,2)));
        maxY = ceil(max(cornersGlobal(:,2)));

        for xi = minX:maxX
            for yi = minY:maxY
                dx = xi - centreX;
                dy = yi - centreY;
                local = R' * [dx; dy];  % inverse rotation
    
                % Check if point lies inside the robot rectangle
                if abs(local(1)) <= halfL && abs(local(2)) <= halfW
                    if maze(yi, xi) == 1
                        crash = true;
                        assignin('base', 'simulationParams', simulationParams);
                    end
                end
            end
        end
    else
        crash = true;
        assignin('base', 'simulationParams', simulationParams);
    end
    if x > 200 * (endBlock(1) - 1) && x < 200 * endBlock(1) && y > 200 * (endBlock(2) - 1) && y < 200 * (endBlock(2))
        if endTime == 0
            endTime = currentTime;
            simulationParams.finishTime = endTime - startTime;
        end
    end
    if x < 200 && y < 200
        startTime = currentTime;
        endTime = 0;
    end
    if test
        simulationParams.sen_noise_line = weight(1);
        simulationParams.sen_noise_dist = weight(2);
        simulationParams.sen_drift = weight(3);
        simulationParams.sen_fail_line = weight(4);
        simulationParams.sen_fail_dist = weight(5);
        simulationParams.sen_fail_var = weight(6);
        simulationParams.com_delay = weight(7);
        simulationParams.whe_slip = weight(8);
    end
end
